simulink model "PDdecoupleCopy02"  (R2021b)
settings: Solver=FixedStepAuto  StartTime=0.0  StopTime=6  FixedStep=1e-3  MaxStep=1e-2  RelTol=1e-5  AbsTol=1e-6
values from neighbouring files (symbols this model uses):
  gravity = [0;0;-g]    [parameters.m]
  Inertia = [5.5*10^(-7) 0 0;0 5.5*10^(-7) 0;0 0 11*10^(-7)]    [parameters.m]
  kd = 9    [parameters.m]
  kp = 30    [parameters.m]
  kq = 250    [parameters.m]
  kw = 6    [parameters.m]
  limite_torque = Inertia*[10;10;10]    [parameters.m]
  Lower_Limit_acc = [-maxacc;-maxacc;-g]    [parameters.m]
  mass = 0.027    [parameters.m]
  MaxThrust = 60*1e-3*9.81    (= 0.5886)    [parameters.m]
  Upper_Limit_acc = [maxacc;maxacc;2*g]    [parameters.m]
libraries: simulink x3
settings Model: Creator=thinkpad  LastModifiedBy=thinkpad

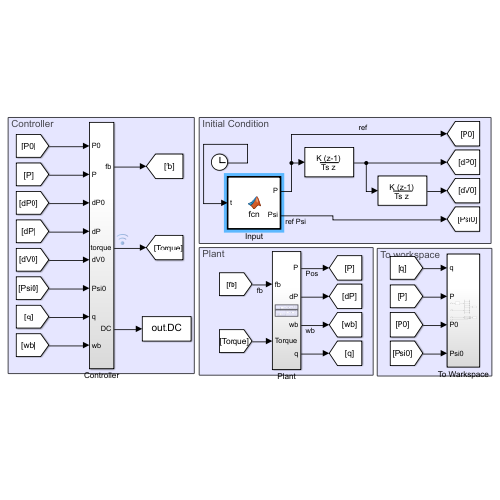
[thumbnail: Simulink's stored preview of the top-level diagram]
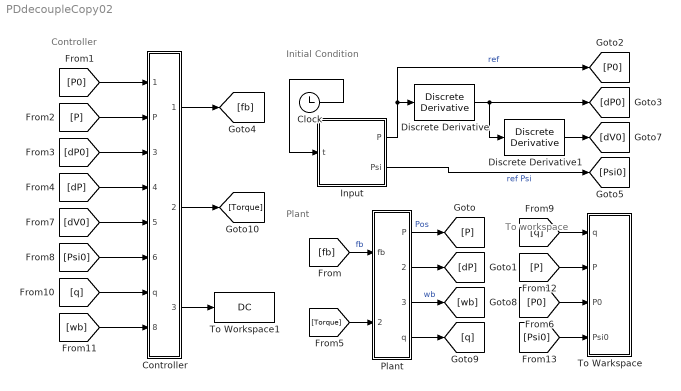
== system PDdecoupleCopy02 ==
  note: To workspace
  note: Controller
  note: Initial Condition
  note: Plant
  Clock : Clock
  Controller : Subsystem
  Discrete Derivative : simulink/Discrete/Discrete Derivative  gainval=1.0  ICPrevScaledInput=0.0  OutMin=[]  OutMax=[]  OutDataType=fixdt(1, 16)  OutScaling=2^-10  DoSatur=off
  Discrete Derivative1 : simulink/Discrete/Discrete Derivative  gainval=1.0  ICPrevScaledInput=0.0  OutMin=[]  OutMax=[]  OutDataType=fixdt(1, 16)  OutScaling=2^-10  DoSatur=off
  Input : MATLAB Function  TreatAsAtomicUnit=on
  Plant : Subsystem
  To Warkspace : Subsystem
  To Workspace1 : ToWorkspace  VariableName=DC  SaveFormat=Timeseries  SampleTime=-1
  wires:
  [Psi0] -> Controller/6(Psi0)
  [wb] -> Controller/8(wb)
  Plant/3(wb) -> [wb]  "wb"
  Plant/2(dP) -> [dP]
  Plant/4(q) -> [q]
  Input/1(P) -> [P0], Discrete Derivative/1  "ref"
  Input/2(Psi) -> [Psi0]  "ref Psi"
  [Torque] -> Plant/2(Torque)
  [fb] -> Plant/1(fb)  "fb"
  Plant/1(P) -> [P]  "Pos"
  Controller/2(torque) -> [Torque]
  Controller/3(DC) -> To Workspace1/1
  [q] -> Controller/7(q)
  [P0] -> Controller/1(P0)
  [dP] -> Controller/4(dP)
  [P] -> Controller/2(P)
  [dV0] -> Controller/5(dV0)
  [dP0] -> Controller/3(dP0)
  Controller/1(fb) -> [fb]
  Clock/1 -> Input/1(t)
  Discrete Derivative1/1 -> [dV0]
  Discrete Derivative/1 -> [dP0], Discrete Derivative1/1
  [q] -> To Warkspace/1(q)
  [P] -> To Warkspace/2(P)
  [P0] -> To Warkspace/3(P0)
  [Psi0] -> To Warkspace/4(Psi0)

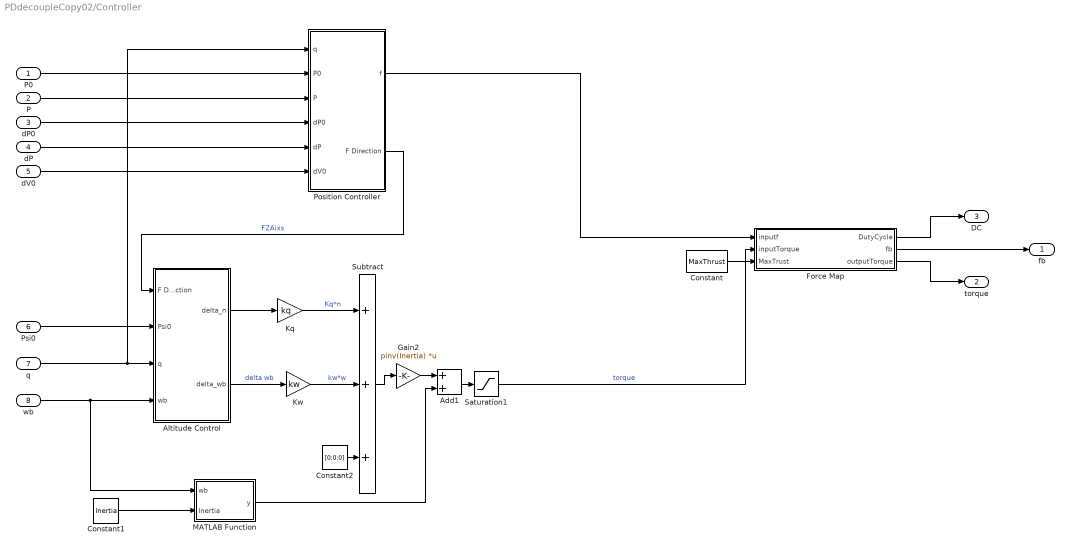
== system PDdecoupleCopy02/Controller ==
  P0 : Inport
  P : Inport  Port=2
  dP0 : Inport  Port=3
  dP : Inport  Port=4
  dV0 : Inport  Port=5
  Psi0 : Inport  Port=6
  q : Inport  Port=7
  wb : Inport  Port=8
  Add1 : Sum
  Altitude Control : Subsystem
  Constant : Constant  Value=MaxThrust
  Constant1 : Constant  Value=Inertia
  Constant2 : Constant  Value=[0;0;0]
  Force Map : MATLAB Function  TreatAsAtomicUnit=on
  Gain2 : Gain  Gain=pinv(Inertia)  Multiplication=Matrix(K*u)
  Kq : Gain  Gain=kq
  Kw : Gain  Gain=kw
  MATLAB Function : MATLAB Function  TreatAsAtomicUnit=on
  Position Controller : Subsystem
  Saturation1 : Saturate  UpperLimit=limite_torque  LowerLimit=-limite_torque
  Subtract : Sum  Inputs=+++
  fb : Outport
  torque : Outport  Port=2
  DC : Outport  Port=3
  wires:
  Kw/1 -> Subtract/2  "kw*w"
  Altitude Control/1(delta_n) -> Kq/1
  Subtract/1 -> Gain2/1
  wb/1 -> MATLAB Function/1(wb), Altitude Control/4(wb)
  q/1 -> Position Controller/1(q), Altitude Control/3(q)
  Altitude Control/2(delta_wb) -> Kw/1  "delta wb"
  Constant2/1 -> Subtract/3
  Add1/1 -> Saturation1/1
  Gain2/1 -> Add1/1
  P/1 -> Position Controller/3(P)
  Kq/1 -> Subtract/1  "Kq*n"
  P0/1 -> Position Controller/2(P0)
  Position Controller/2(F Direction) -> Altitude Control/1(F Direction)  "FZAixs"
  Psi0/1 -> Altitude Control/2(Psi0)
  dV0/1 -> Position Controller/6(dV0)
  dP0/1 -> Position Controller/4(dP0)
  dP/1 -> Position Controller/5(dP)
  Constant/1 -> Force Map/3(MaxTrust)
  Saturation1/1 -> Force Map/2(inputTorque)  "torque"
  Force Map/2(fb) -> fb/1
  Force Map/3(outputTorque) -> torque/1
  Force Map/1(DutyCycle) -> DC/1
  Position Controller/1(f) -> Force Map/1(inputf)
  Constant1/1 -> MATLAB Function/2(Inertia)
  MATLAB Function/1(y) -> Add1/2

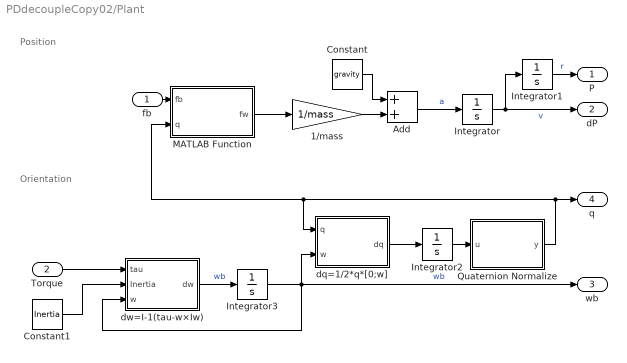
== system PDdecoupleCopy02/Plant ==
  note: Orientation
  note: Position
  fb : Inport
  Torque : Inport  Port=2  PortDimensions=3
  1/mass : Gain  Gain=1/mass
  Add : Sum
  Constant : Constant  Value=gravity
  Constant1 : Constant  Value=Inertia
  Integrator : Integrator  InitialCondition=[0;0;0]
  Integrator1 : Integrator  InitialCondition=[0;0;0]
  Integrator2 : Integrator  InitialCondition=[1;0;0;0]
  Integrator3 : Integrator  InitialCondition=[0;0;0]
  MATLAB Function : MATLAB Function  TreatAsAtomicUnit=on
  Quaternion Normalize : MATLAB Function  TreatAsAtomicUnit=on
  dq=1/2*q*[0;w] : MATLAB Function  TreatAsAtomicUnit=on
  dw=I-1(tau-w×Iw) : MATLAB Function  TreatAsAtomicUnit=on
  P : Outport
  dP : Outport  Port=2
  wb : Outport  Port=3
  q : Outport  Port=4
  wires:
  Integrator1/1 -> P/1  "r"
  Constant/1 -> Add/1
  Integrator/1 -> Integrator1/1, dP/1  "v"
  Add/1 -> Integrator/1  "a"
  Quaternion Normalize/1(y) -> MATLAB Function/2(q), dq=1/2*q*[0;w]/1(q), q/1
  dq=1/2*q*[0;w]/1(dq) -> Integrator2/1
  Integrator2/1 -> Quaternion Normalize/1(u)
  1/mass/1 -> Add/2
  MATLAB Function/1(fw) -> 1/mass/1
  fb/1 -> MATLAB Function/1(fb)
  Constant1/1 -> dw=I-1(tau-w×Iw)/2(Inertia)
  Torque/1 -> dw=I-1(tau-w×Iw)/1(tau)
  Integrator3/1 -> dw=I-1(tau-w×Iw)/3(w), wb/1, dq=1/2*q*[0;w]/2(w)  "wb"
  dw=I-1(tau-w×Iw)/1(dw) -> Integrator3/1  "wb"

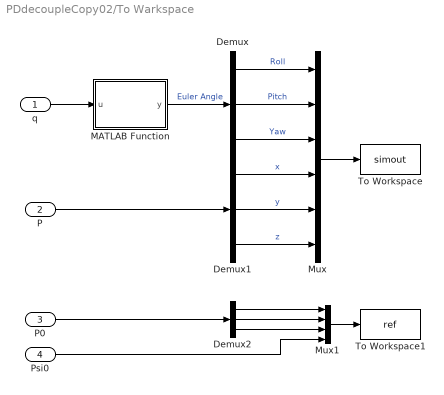
== system PDdecoupleCopy02/To Warkspace ==
  q : Inport
  P : Inport  Port=2
  P0 : Inport  Port=3
  Psi0 : Inport  Port=4
  Demux : Demux  Outputs=3
  Demux1 : Demux  Outputs=3
  Demux2 : Demux  Outputs=3
  MATLAB Function : MATLAB Function  TreatAsAtomicUnit=on
  Mux : Mux  Inputs=6
  Mux1 : Mux
  To Workspace : ToWorkspace  VariableName=simout  SampleTime=-1
      settings: Save2DSignal=2-D array (concatenate along first dimension)
  To Workspace1 : ToWorkspace  VariableName=ref  SampleTime=-1
      settings: Save2DSignal=2-D array (concatenate along first dimension)
  wires:
  Demux1/3 -> Mux/6  "z"
  Mux/1 -> To Workspace/1
  Demux1/2 -> Mux/5  "y"
  Demux1/1 -> Mux/4  "x"
  MATLAB Function/1(y) -> Demux/1  "Euler Angle"
  q/1 -> MATLAB Function/1(u)
  P/1 -> Demux1/1
  P0/1 -> Demux2/1
  Demux2/1 -> Mux1/1
  Demux2/2 -> Mux1/2
  Demux2/3 -> Mux1/3
  Psi0/1 -> Mux1/4
  Mux1/1 -> To Workspace1/1
  Demux/1 -> Mux/1  "Roll"
  Demux/2 -> Mux/2  "Pitch"
  Demux/3 -> Mux/3  "Yaw"

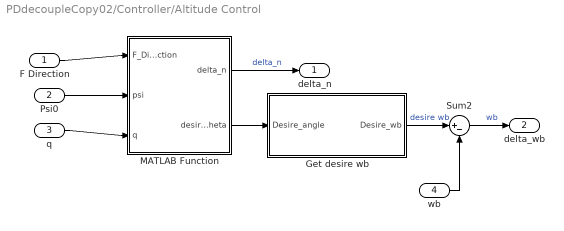
== system PDdecoupleCopy02/Controller/Altitude Control ==
  F Direction : Inport
  Psi0 : Inport  Port=2
  q : Inport  Port=3
  wb : Inport  Port=4
  Get desire wb : Subsystem
  MATLAB Function : MATLAB Function  TreatAsAtomicUnit=on
  Sum2 : Sum  Inputs=|+-
  delta_n : Outport
  delta_wb : Outport  Port=2
  wires:
  q/1 -> MATLAB Function/3(q)
  Sum2/1 -> delta_wb/1  "wb"
  wb/1 -> Sum2/2
  Get desire wb/1(Desire_wb) -> Sum2/1  "desire wb"
  MATLAB Function/1(delta_n) -> delta_n/1  "delta_n"
  Psi0/1 -> MATLAB Function/2(psi)
  F Direction/1 -> MATLAB Function/1(F_Direction)
  MATLAB Function/2(desire_Theta) -> Get desire wb/1(Desire_angle)

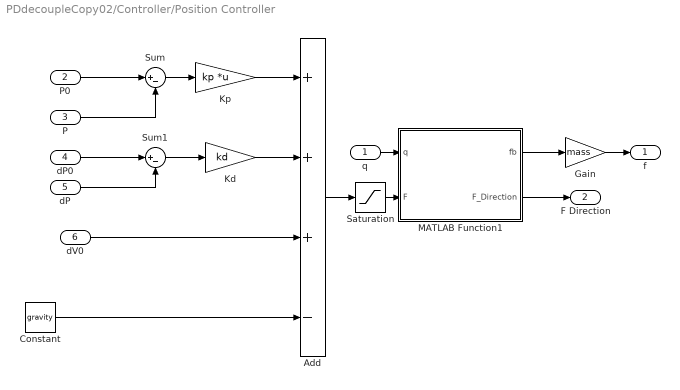
== system PDdecoupleCopy02/Controller/Position Controller ==
  q : Inport
  P0 : Inport  Port=2
  P : Inport  Port=3
  dP0 : Inport  Port=4
  dP : Inport  Port=5
  dV0 : Inport  Port=6
  Add : Sum  Inputs=+++-
  Constant : Constant  Value=gravity
  Gain : Gain  Gain=mass
  Kd : Gain  Gain=kd
  Kp : Gain  Gain=kp  Multiplication=Matrix(K*u)
  MATLAB Function1 : MATLAB Function  TreatAsAtomicUnit=on
  Saturation : Saturate  UpperLimit=Upper_Limit_acc  LowerLimit=Lower_Limit_acc
  Sum : Sum  Inputs=|+-
  Sum1 : Sum  Inputs=|+-
  f : Outport
  F Direction : Outport  Port=2
  wires:
  P/1 -> Sum/2
  Kp/1 -> Add/1
  dP/1 -> Sum1/2
  Sum/1 -> Kp/1
  Sum1/1 -> Kd/1
  Kd/1 -> Add/2
  q/1 -> MATLAB Function1/1(q)
  dP0/1 -> Sum1/1
  dV0/1 -> Add/3
  P0/1 -> Sum/1
  Gain/1 -> f/1
  Add/1 -> Saturation/1
  Saturation/1 -> MATLAB Function1/2(F)
  MATLAB Function1/2(F_Direction) -> F Direction/1
  Constant/1 -> Add/4
  MATLAB Function1/1(fb) -> Gain/1

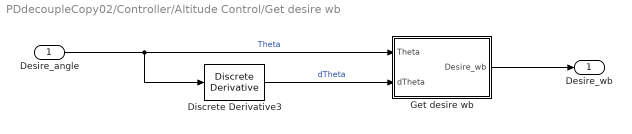
== system PDdecoupleCopy02/Controller/Altitude Control/Get desire wb ==
  Desire_angle : Inport
  Discrete Derivative3 : simulink/Discrete/Discrete Derivative  gainval=1.0  ICPrevScaledInput=0.0  OutMin=[]  OutMax=[]  OutDataType=fixdt(1, 16)  OutScaling=2^-10  DoSatur=off
  Get desire wb : MATLAB Function  TreatAsAtomicUnit=on
  Desire_wb : Outport
  wires:
  Discrete Derivative3/1 -> Get desire wb/2(dTheta)  "dTheta"
  Desire_angle/1 -> Discrete Derivative3/1, Get desire wb/1(Theta)  "Theta"
  Get desire wb/1(Desire_wb) -> Desire_wb/1

== matlab function PDdecoupleCopy02/To Warkspace/MATLAB Function ==
  data: u input size=4; y output size=3
function y = fcn(u)
coder.extrinsic("quat2angle");
y=zeros(3,1);
[y(3),y(2),y(1)]=quat2angle(u');
end

== matlab function PDdecoupleCopy02/Controller/Altitude Control/Get desire wb/Get desire wb ==
  data: Theta input size=3; Desire_wb output size=3; dTheta input size=3
function Desire_wb = T_dTheta(Theta, dTheta)
row=Theta(1);
pitch=Theta(2);
yaw=Theta(3);
T=[cos(yaw)*cos(pitch) -sin(yaw) 0;
    cos(pitch)*sin(yaw) cos(yaw) 0;
    -sin(pitch) 0 1];
Desire_wb=T*dTheta;
end

== matlab function PDdecoupleCopy02/Input ==
  data: t input size=1; P output size=3; Psi output size=1
function [P, Psi] = fcn(t)
P=[sin(t)*0.2;sin(t)*0.2;sin(t)*0.2];
Psi=sin(t)*0.5;
end

== matlab function PDdecoupleCopy02/Plant/dq=1//2*q*[0;w] ==
  data: q input; dq output; w input
function dq = q2dq(q,w)
dq=1/2*UnitQuatMultiply(q,[0;w]);
end

== matlab function PDdecoupleCopy02/Controller/Altitude Control/MATLAB Function ==
  data: delta_n output size=3; F_Direction input size=3; psi input size=1; q input size=4; desire_Theta output
function [delta_n, desire_Theta] = fcn(F_Direction, psi, q)
coder.extrinsic('dcm2angle');
coder.extrinsic('dcm2quat');


    u3=F_Direction;
    u1=[cos(psi);sin(psi);0];
    u2=cross(u3,u1);
    u2=u2/norm(u2);
    u1=cross(u2,u3);
    u1=u1/norm(u1);
    R=[u1 u2 u3];
    
    q0=DCM2UnitQuat(R);



    desire_Theta=zeros(3,1);
    [desire_Theta(1),desire_Theta(2),desire_Theta(3)]=dcm2angle(R');


    delta_q=UnitQuatMultiply(q0,UnitQuatAdjugate(q));
    delta_n=delta_q(2:4);
end

== matlab function PDdecoupleCopy02/Controller/Position Controller/MATLAB Function1 ==
  data: q input size=4; fb output size=1; F input size=3; F_Direction output size=3
function [fb, F_Direction] = fcn(q, F)

F_Direction=F/(norm(F));
fb=F'*UnitQuatRotation(q,[0;0;1]);
end

== matlab function PDdecoupleCopy02/Controller/Force Map ==
  data: inputf input size=1; DutyCycle output size=4; inputTorque input size=3; MaxTrust input size=1; fb output size=1; outputTorque output size=3
function [DutyCycle,fb,outputTorque] =ForceMap(inputf,inputTorque,MaxTrust)

TransMatrix=[1 1 1 1;
    -0.0046 -0.0046 0.0046 0.0046;
    -0.0046 0.0046 0.0046 -0.0046;
    -0.005964552  0.005964552  -0.005964552  0.005964552];%%%%%%%%%%%%
u=[inputf;inputTorque];

f=TransMatrix\u;


%% f>=0
for i=1:4
    if f(i)<0
        f(i)=0;
    end
end


%% f<=f_Max

scale=[1 1 1 1]*f;


if scale>MaxTrust
    f=f/scale*MaxTrust;
end

u=TransMatrix*f;
fb=u(1);
outputTorque=u(2:4);
DutyCycle=Thrust2PWM(f);
end

%%
function dc=Thrust2PWM(f)

% %http://mikehamer.info/assets/papers/Crazyflie%20Modelling.pdf

% a=2.130295*1e-11;
% b=1.032633*1e-6;


a=6.1923723*1e-9;
b=5.467*1e-4;
% c=-0.099-f;
dc=zeros(4,1);


    for i=1:4
        c=-0.099-f(i)/9.81*1e3;
        dc(i)=(-b+sqrt(b^2-4*a*c))/(2*a);
        dc(i)=floor(dc(i))+1;
       
    end
end
%%

== matlab function PDdecoupleCopy02/Plant/dw=I-1(tau-w×Iw) ==
  data: tau input; dw output; Inertia input; w input
function dw = fcn(tau,Inertia,w)
dw=pinv(Inertia)*(tau-cross(w,Inertia*w));
end

== matlab function PDdecoupleCopy02/Controller/MATLAB Function ==
  data: wb input; y output; Inertia input
function y = fcn(wb,Inertia)

y=cross(wb,Inertia*wb);

== matlab function PDdecoupleCopy02/Plant/MATLAB Function ==
  data: fb input size=1; q input size=4; fw output size=3
function fw = BodyToWorld(fb,q)
% fb is the Thrust, scalar
% q is the Orientation representing by Quaternion
fw=UnitQuatRotation(q,[0;0;fb]);
end

== matlab function PDdecoupleCopy02/Plant/Quaternion Normalize ==
  data: u input; y output
function y = QuatNormalize(u)
y=QuaternionNormalize(u);
end
